simulink model "series_inverter"  (R2023b)
settings: Solver=VariableStepAuto  StartTime=0.0  StopTime=0.03  RelTol=1e-3
libraries: spsSeriesRLCBranchLib x5, spsThyristorLib x2, spsVoltageMeasurementLib x2, spsDCVoltageSourceLib x1, spsLinearTransformerLib x1, sps_lib x1
settings Model: Creator=10bah  LastModifiedBy=10bah

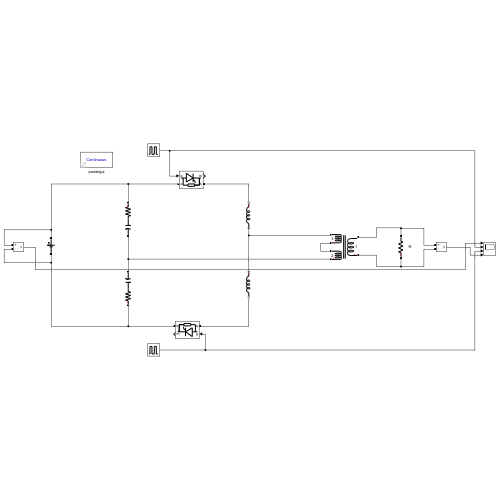
[thumbnail: Simulink's stored preview of the top-level diagram]
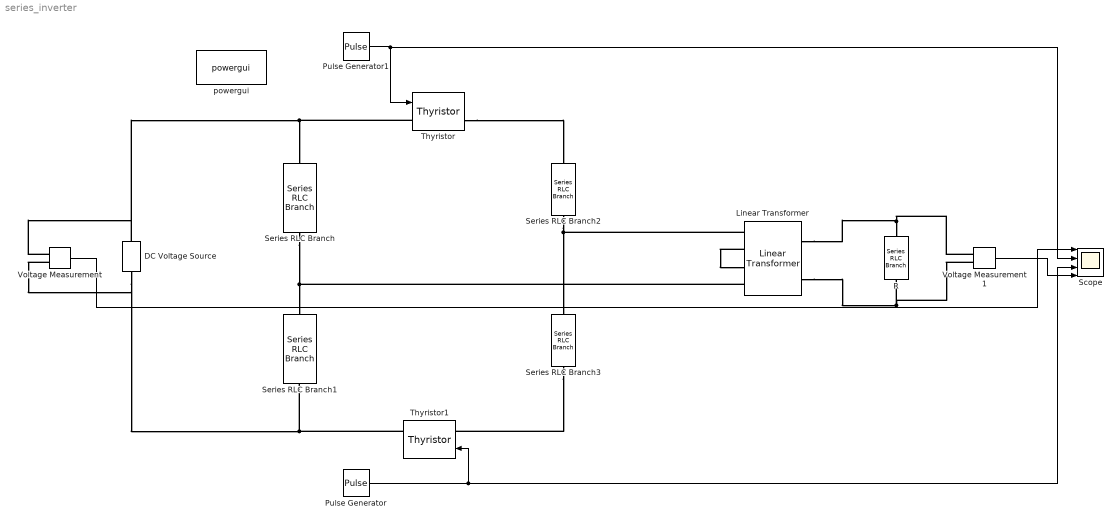
== system series_inverter ==
  DC Voltage Source : spsDCVoltageSourceLib/DC Voltage Source  Amplitude=13.5  Measurements=None
  Linear Transformer : spsLinearTransformerLib/Linear Transformer  UNITS=pu  NominalPower=[ 250e6 60 ]  winding1="[ 735e3  0.002  0.08 ]"  winding2="[ 315e3  0.002  0.08 ]"  ThreeWindings=on  winding3=[ 315e3 0.002 0.08 ]  RmLm=[ 500 500 ]  Measurements=None  DataType=off
  Pulse Generator : DiscretePulseGenerator  PulseType=Time based  Period=0.02  PulseWidth=5  PhaseDelay=0.0133
  Pulse Generator1 : DiscretePulseGenerator  PulseType=Time based  Period=0.02  PulseWidth=5  PhaseDelay=0.0033
  R : spsSeriesRLCBranchLib/Series RLC Branch  LConnTagsString=__new0  RConnTagsString=__new0  BranchType=R  Resistance=5  Inductance=1e-3  SetiL0=off  InitialCurrent=0  Capacitance=1e-6  Setx0=off  InitialVoltage=0  Measurements=None
  Scope : Scope  NumInputPorts=4
  Series RLC Branch : spsSeriesRLCBranchLib/Series RLC Branch  LConnTagsString=__new0  RConnTagsString=__new0  BranchType=RC  Resistance=10  Inductance=1e-3  SetiL0=off  InitialCurrent=0  Capacitance=10e-6  Setx0=off  InitialVoltage=0  Measurements=None
  Series RLC Branch1 : spsSeriesRLCBranchLib/Series RLC Branch  LConnTagsString=__new0  RConnTagsString=__new0  BranchType=RC  Resistance=10  Inductance=1e-3  SetiL0=off  InitialCurrent=0  Capacitance=10e-6  Setx0=off  InitialVoltage=0  Measurements=None
  Series RLC Branch2 : spsSeriesRLCBranchLib/Series RLC Branch  LConnTagsString=__new0  RConnTagsString=__new0  BranchType=L  Resistance=1  Inductance=4.2e-3  SetiL0=off  InitialCurrent=0  Capacitance=1e-6  Setx0=off  InitialVoltage=0  Measurements=None
  Series RLC Branch3 : spsSeriesRLCBranchLib/Series RLC Branch  LConnTagsString=__new0  RConnTagsString=__new0  BranchType=L  Resistance=1  Inductance=4.2e-3  SetiL0=off  InitialCurrent=0  Capacitance=1e-6  Setx0=off  InitialVoltage=0  Measurements=None
  Thyristor : spsThyristorLib/Thyristor  Ron=0.001  Lon=0  Vf=0.8  IC=0  Rs=500  Cs=250e-9  Measurements=on
  Thyristor1 : spsThyristorLib/Thyristor  Ron=0.001  Lon=0  Vf=0.8  IC=0  Rs=500  Cs=250e-9  Measurements=on
  Voltage Measurement : spsVoltageMeasurementLib/Voltage Measurement  PhasorSimulation=off  OutputType=Complex  PSBequivalent=0
  Voltage Measurement1 : spsVoltageMeasurementLib/Voltage Measurement  PhasorSimulation=off  OutputType=Complex  PSBequivalent=0
  powergui : sps_lib/powergui  Priority=1  SimulationMode=Continuous  SampleTime=50e-6  frequency=60  Iterations=50  frequencyindice=0  Pbase=100e6  ErrMax=1e-4  UnitsV=kV  UnitsW=MW  buscounter=0  FunctionMessages=off  echomessages=off  EnableUseOfTLC=off  CurrentSourceSwitches=off  DisableSnubberDevices=off  DisableRonSwitches=off  DisableVfSwitches=off  DisplayEquations=off  AutomaticDiscreteSolvers=off  SolverType=Tustin/Backward Euler (TBE)  Interpol=off  ExternalGateDelay=off  methode=off  Ts=100  x0status=blocks  SPID=on  SwTol=0  HookPort=off  NonlinearTolerance=1e-4  nMaxIteration=100  ContinueOnMaxIteration=off  RestoreLinks=warning  ResistiveCurrentMeasurement=off  Frange=[0:2:500]  Ylog=off  Xlog=on  ShowGrid=off  save=off  variable=ZData  structure=0  ZoomFFT=off  StartTime=0.0  cycles=1  DisplayStyle=1  fundamental=60  FreqAxis=off  MaxFrequency=1000  frequencyindicesteady=1  RmsSteady=1  display=off
  wires:
  Pulse Generator1/1 -> Scope/2, Thyristor/1
  Pulse Generator/1 -> Thyristor1/1, Scope/3
  Voltage Measurement/1 -> Scope/1
  Voltage Measurement1/1 -> Scope/4
  connections:
  Thyristor/LConn1 -- Voltage Measurement/LConn1 -- DC Voltage Source/RConn1 -- Series RLC Branch/LConn1
  Series RLC Branch/RConn1 -- Linear Transformer/RConn1 -- Series RLC Branch1/RConn1
  Thyristor1/RConn1 -- Voltage Measurement/LConn2 -- DC Voltage Source/LConn1 -- Series RLC Branch1/LConn1
  Thyristor/RConn1 -- Series RLC Branch2/LConn1
  Series RLC Branch2/RConn1 -- Linear Transformer/RConn4 -- Series RLC Branch3/LConn1
  Series RLC Branch3/RConn1 -- Thyristor1/LConn1
  Linear Transformer/RConn3 -- Linear Transformer/RConn2
  Linear Transformer/LConn2 -- Voltage Measurement1/LConn1 -- R/RConn1
  Linear Transformer/LConn1 -- Voltage Measurement1/LConn2 -- R/LConn1
